simulink model "ActiveSuspensionSim"  (R2022a)
settings: Solver=ode1  StartTime=0.0  StopTime=10.0  FixedStep=0.001  RelTol=1e-3
InitFcn:
  | ActiveSuspensionParameters
  | ActiveSuspensionMenu
StopFcn:
  | ActiveSuspensionSystemAutoGrading
values from neighbouring files (symbols this model uses):
  Active = menu('Active Control is On',                  'Yes',              	'No')    [ActiveSuspensionMenu.m]
  Cs = 350    [ActiveSuspensionParameters.m]    (also in ActiveSuspensionScript.m)
  Cus = 7020    [ActiveSuspensionParameters.m]    (also in ActiveSuspensionScript.m)
  Ks = 40000    [ActiveSuspensionParameters.m]    (also in ActiveSuspensionScript.m)
  Ms = 2900    [ActiveSuspensionParameters.m]    (also in ActiveSuspensionScript.m)
  Mus = 300    [ActiveSuspensionParameters.m]    (also in ActiveSuspensionScript.m)
  Profile = menu('Road profile',                  'Ramp',              	'Sinusoid',                 'Rectified Sinusoid',                 'Random')    [ActiveSuspensionMenu.m]
libraries: simulink x1
settings Model: Creator=burl  LastModifiedBy=prajw
settings SolverCC: AlgebraicLoopSolver=TrustRegion
settings DataIOCC: ReturnWorkspaceOutputs=off
settings DebuggingCC: UnconnectedInputMsg=warning  UnconnectedOutputMsg=warning  UnconnectedLineMsg=warning  PregeneratedLibrarySubsystemCodeDiagnostic=none  SFMachineParentedDataDiag=warning  ArithmeticOperatorsInVariantConditions=warning
settings SFSimCC: SimUseLocalCustomCode=off  CustomCodeUndefinedFunction=UseInterfaceOnly
settings RTWCC: RTWUseLocalCustomCode=off

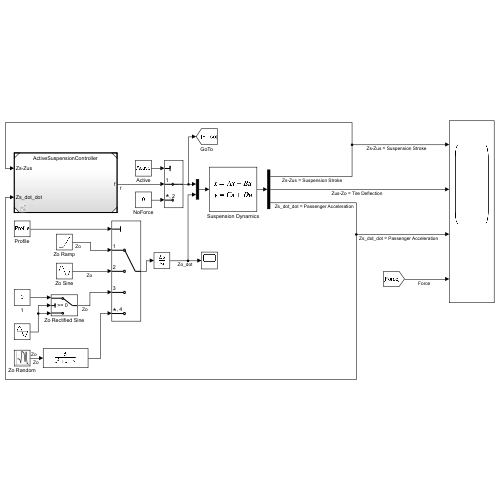
[thumbnail: Simulink's stored preview of the top-level diagram]
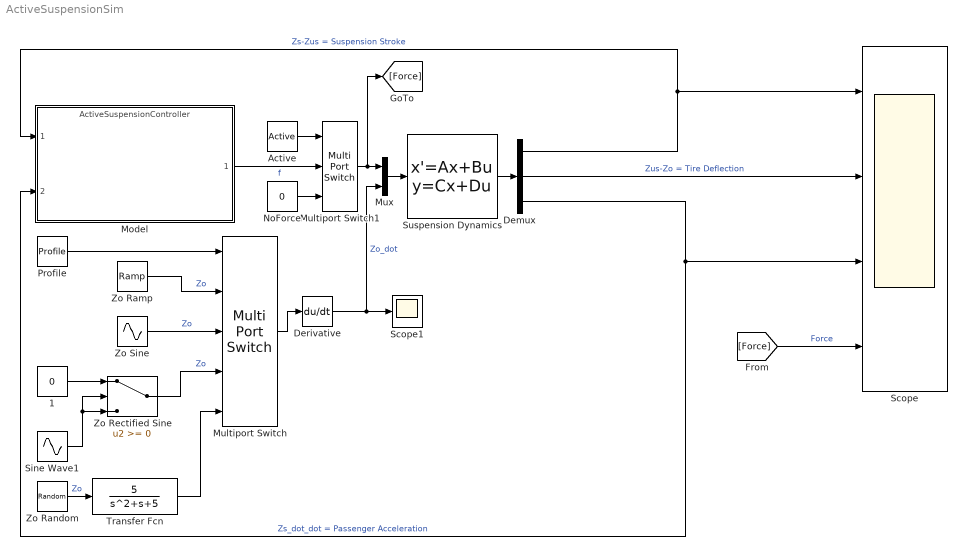
== system ActiveSuspensionSim ==
  1 : Constant  Value=0
  Active : Constant  Value=Active
  Demux : Demux  Outputs=3
  Derivative : Derivative
  Model : ModelReference  ModelNameDialog=ActiveSuspensionController  SimulationMode=Normal  ModelReferenceVersion=9.3
  Multiport Switch : MultiPortSwitch  Inputs=4  SaturateOnIntegerOverflow=off  InputSameDT=off
  Multiport Switch1 : MultiPortSwitch  Inputs=2  SaturateOnIntegerOverflow=off  InputSameDT=off
  Mux : Mux  Inputs=2
  NoForce : Constant  Value=0
  Profile : Constant  Value=Profile
  Scope : Scope  NumInputPorts=4
  Scope1 : Scope
  Sine Wave1 : Sin  Amplitude=0.05  Frequency=pi  SampleTime=0
  Suspension Dynamics : StateSpace  A=|  B=[0 -1 ; 1/Mus Cus/Mus ; 0 0 ;-1/Ms 0]  C=[0 0 1 0 ; 1 0 0 0 ; 0 Cs/Ms -Ks/Ms -Cs/Ms]  D=[0 0 ; 0 0 ; 0 0]  InitialCondition=0
      | [ 0 1 0 0 ; -Kus/Mus -(Cs+Cus)/Mus Ks/Mus Cs/Mus ; 0 -1 0 1 ;
      | 0 Cs/Ms -Ks/Ms -Cs/Ms ]
  Transfer Fcn : TransferFcn  Numerator=[5]  Denominator=[1 1 5]
  Zo Ramp : simulink/Sources/Ramp  slope=0.1  start=1  InitialOutput=0
  Zo Random : RandomNumber  Variance=0.1  SampleTime=0.01
  Zo Rectified Sine : Switch  SaturateOnIntegerOverflow=off  InputSameDT=off
  Zo Sine : Sin  Amplitude=0.05  Frequency=pi  SampleTime=0
  wires:
  Model/1 -> Multiport Switch1/2  "f"
  Mux/1 -> Suspension Dynamics/1
  Suspension Dynamics/1 -> Demux/1
  Demux/1 -> Model/1, Scope/1  "Zs-Zus = Suspension Stroke"
  Demux/3 -> Scope/3, Model/2  "Zs_dot_dot = Passenger Acceleration"
  Sine Wave1/1 -> Zo Rectified Sine/2, Zo Rectified Sine/3
  1/1 -> Zo Rectified Sine/1
  Zo Sine/1 -> Multiport Switch/3  "Zo"
  Multiport Switch/1 -> Derivative/1
  Zo Rectified Sine/1 -> Multiport Switch/4  "Zo"
  Zo Ramp/1 -> Multiport Switch/2  "Zo"
  Profile/1 -> Multiport Switch/1
  Derivative/1 -> Scope1/1, Mux/2  "Zo_dot"
  Demux/2 -> Scope/2  "Zus-Zo = Tire Deflection"
  [Force] -> Scope/4  "Force"
  Multiport Switch1/1 -> [Force], Mux/1
  Active/1 -> Multiport Switch1/1
  NoForce/1 -> Multiport Switch1/3
  Zo Random/1 -> Transfer Fcn/1  "Zo"
  Transfer Fcn/1 -> Multiport Switch/5
